simulink model "PardoMuxTwo"  (R2023b)
settings: Solver=VariableStepAuto  StartTime=0.0  StopTime=10.0  RelTol=1e-3
settings Model: Creator=jsonm  LastModifiedBy=jsonm

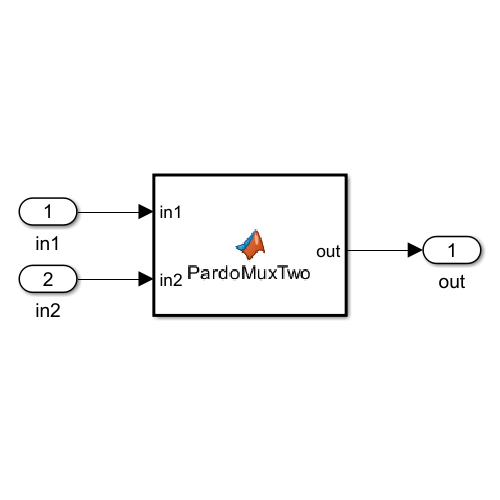
[thumbnail: Simulink's stored preview of the top-level diagram]
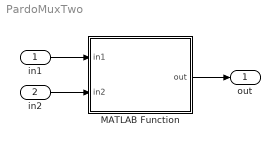
== system PardoMuxTwo ==
  in1 : Inport
  in2 : Inport  Port=2
  MATLAB Function : MATLAB Function  TreatAsAtomicUnit=on
  out : Outport
  wires:
  in1/1 -> MATLAB Function/1(in1)
  in2/1 -> MATLAB Function/2(in2)
  MATLAB Function/1(out) -> out/1

== matlab function PardoMuxTwo/MATLAB Function ==
  data: in1 input; out output; in2 input
function out = PardoMuxTwo(in1, in2)
% Method to mux one of two possible inputs into one output based on assumption
% that processes run in parallel and must all complete.
%
% Non-valid output is negative
%
% Written by: Darian Muresan
% Modified by: Jason McCauley

if nargin < 1
        in1 = -1;
        in2 = -1;
elseif nargin < 2
        in2 = -1;
end

inVector = [in1, in2];
validInputs = inVector(inVector > 0); % Only select positive inputs

if isempty(validInputs)
        out = -1; 
else
        out = max(validInputs);
end
